simulink model "BASK"  (R2016a)
settings: Solver=VariableStepAuto  StartTime=0.0  StopTime=10.0  RelTol=1e-3
libraries: dsparch4 x2, commrandsrc3 x1, commsink2 x1
settings Model: Creator=hp  LastModifiedBy=hp

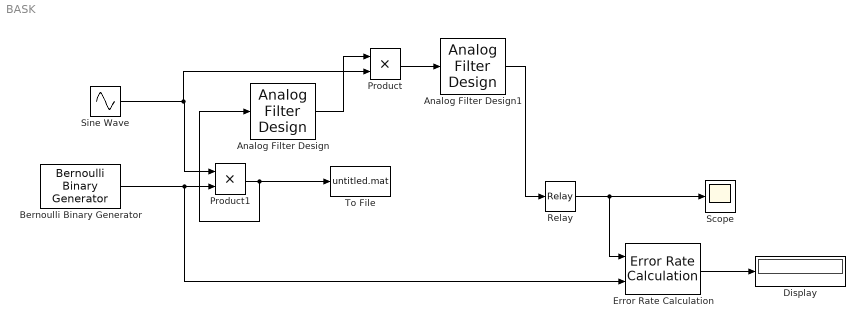
== system BASK ==
  Analog Filter Design : dsparch4/Analog Filter Design  method=Butterworth  filttype=Bandpass  N=1  Wlo=1800*pi  Whi=2200*pi  Rp=2  Rs=40
  Analog Filter Design1 : dsparch4/Analog Filter Design  method=Butterworth  filttype=Lowpass  N=2  Wlo=200*pi  Whi=80  Rp=2  Rs=40
  Bernoulli Binary Generator : commrandsrc3/Bernoulli Binary Generator  ProbabilityOfZero=0.5  SeedSource=Parameter  Seed=61  SampleTime=1/100  SamplesPerFrame=1  OutputDataType=double  SimulateUsing=Interpreted execution
  Display : Display
  Error Rate Calculation : commsink2/Error Rate Calculation  N=0  st_delay=0  cp_mode=Entire frame  subframe=[]  PMode=Port  WsName=ErrorVec  RsMode2=off  stop=off  numErr=100  maxBits=1e6
  Product : Product
  Product1 : Product
  Relay : Relay  OnSwitchValue=0.25  OffSwitchValue=0.25
  Scope : Scope
  Sine Wave : Sin  Frequency=2000*pi  SampleTime=1/10000
  To File : ToFile  SaveFormat=Timeseries
  wires:
  Bernoulli Binary Generator/1 -> Error Rate Calculation/2, Product1/2
  Product1/1 -> Analog Filter Design/1, To File/1
  Product/1 -> Analog Filter Design1/1
  Analog Filter Design1/1 -> Relay/1
  Relay/1 -> Error Rate Calculation/1, Scope/1
  Error Rate Calculation/1 -> Display/1
  Sine Wave/1 -> Product/2, Product1/1
  Analog Filter Design/1 -> Product/1
